simulink model "led_last_press_model"  (R2025a)
settings: Solver=FixedStepDiscrete  StartTime=0.0  StopTime=10  FixedStep=1  RelTol=1e-3
libraries: simulink x3
settings Model: Creator=mahij  LastModifiedBy=mahij

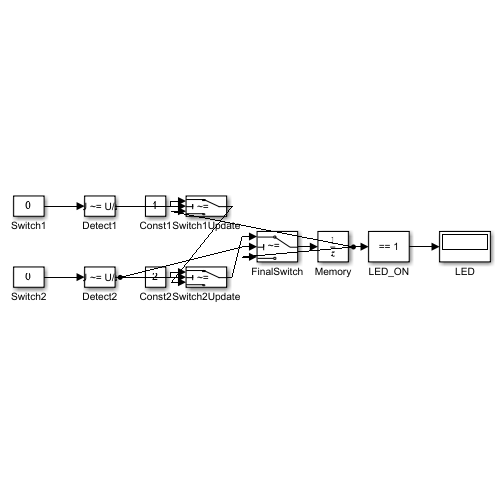
[thumbnail: Simulink's stored preview of the top-level diagram]
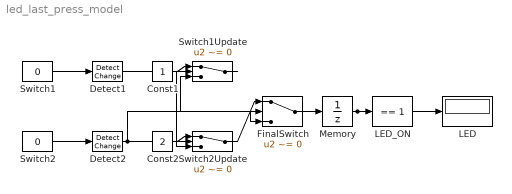
== system led_last_press_model ==
  Const1 : Constant
  Const2 : Constant  Value=2
  Detect1 : simulink/Logic and Bit Operations/Detect Change  vinit=0  OutDataTypeStr=boolean
  Detect2 : simulink/Logic and Bit Operations/Detect Change  vinit=0  OutDataTypeStr=boolean
  FinalSwitch : Switch  Criteria=u2 ~= 0  Threshold=0.5  SaturateOnIntegerOverflow=off  InputSameDT=off
  LED : Display
  LED_ON : simulink/Logic and Bit Operations/Compare To Constant  relop===  const=1  OutDataTypeStr=boolean
  Memory : UnitDelay  HasFrameUpgradeWarning=on
  Switch1 : Constant  Value=0
  Switch1Update : Switch  Criteria=u2 ~= 0  Threshold=0.5  SaturateOnIntegerOverflow=off  InputSameDT=off
  Switch2 : Constant  Value=0
  Switch2Update : Switch  Criteria=u2 ~= 0  Threshold=0.5  SaturateOnIntegerOverflow=off  InputSameDT=off
  wires:
  Switch1/1 -> Detect1/1
  Switch2/1 -> Detect2/1
  Const1/1 -> Switch1Update/1
  Detect1/1 -> Switch1Update/2
  Memory/1 -> Switch1Update/3, FinalSwitch/3, LED_ON/1
  Const2/1 -> Switch2Update/1
  Detect2/1 -> Switch2Update/2, FinalSwitch/2
  Switch1Update/1 -> Switch2Update/3
  Switch2Update/1 -> FinalSwitch/1
  FinalSwitch/1 -> Memory/1
  LED_ON/1 -> LED/1
